simulink model "main_vehicle_model"  (R2023b)
settings: Solver=FixedStepAuto  StartTime=0.0  StopTime=999  RelTol=1e-3  EnableMultiTasking=on
libraries: mbedblockslib x22, mcbcontrolslib x3, slpidlib x1, raspberrypiIMUsensorslib x1, simulink x1
settings Model: SimulationMode=external  ExtModeTrigDuration=10  Creator=Aidan  LastModifiedBy=Aidan
settings SolverCC: AutoInsertRateTranBlk=on
settings OptimizationCC: EnhancedBackFolding=on  PassReuseOutputArgsAs=Individual arguments  ZeroExternalMemoryAtStartup=off  ZeroInternalMemoryAtStartup=off  MaxStackSize=64  OptimizeBlockOrder=speed  DifferentSizesBufferReuse=on  OptimizationCustomize=off  EfficientTunableParamExpr=on
settings DebuggingCC: ParameterTunabilityLossMsg=error
settings HardwareCC: ProdBitPerPointer=32  ProdBitPerSizeT=32  ProdBitPerPtrDiffT=32  ProdLargestAtomicInteger=Long  ProdLargestAtomicFloat=Double  ProdWordSize=32  ProdLongLongMode=on  ProdHWDeviceType=ARM Compatible->ARM Cortex
settings SFSimCC: MATLABDynamicMemAlloc=off
settings RTWCC: Description=Embedded Coder  SystemTargetFile=ert.tlc  HardwareBoard=STM32 Nucleo F746ZG  TemplateMakefile=ert_default_tmf  Toolchain=GNU Tools for ARM Embedded Processors
settings CodeAppCC: ForceParamTrailComments=on  IgnoreCustomStorageClasses=off  OperatorAnnotations=on  SimulinkDataObjDesc=on  SFDataObjDesc=on  InsertBlockDesc=on
settings ERTTargetCC: SupportContinuousTime=on  ExtMode=on  ExtModeTransport=3  ExtModeStaticAlloc=on  ExtModeStaticAllocSize=2000  ExtModeMexFile=ext_xcp  ExtModeMexArgs=1 10 115200  ExtModeIntrfLevel=Level2 - Open

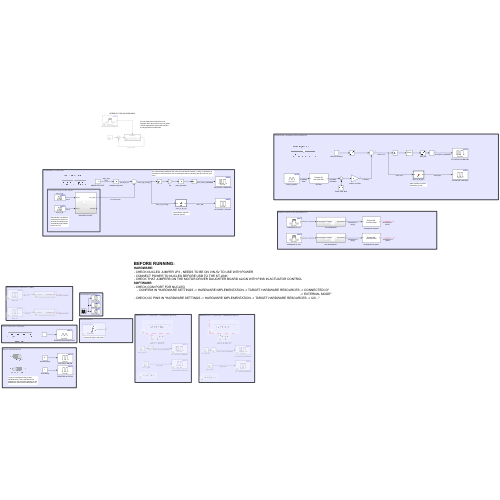
[thumbnail: Simulink's stored preview of the top-level diagram]
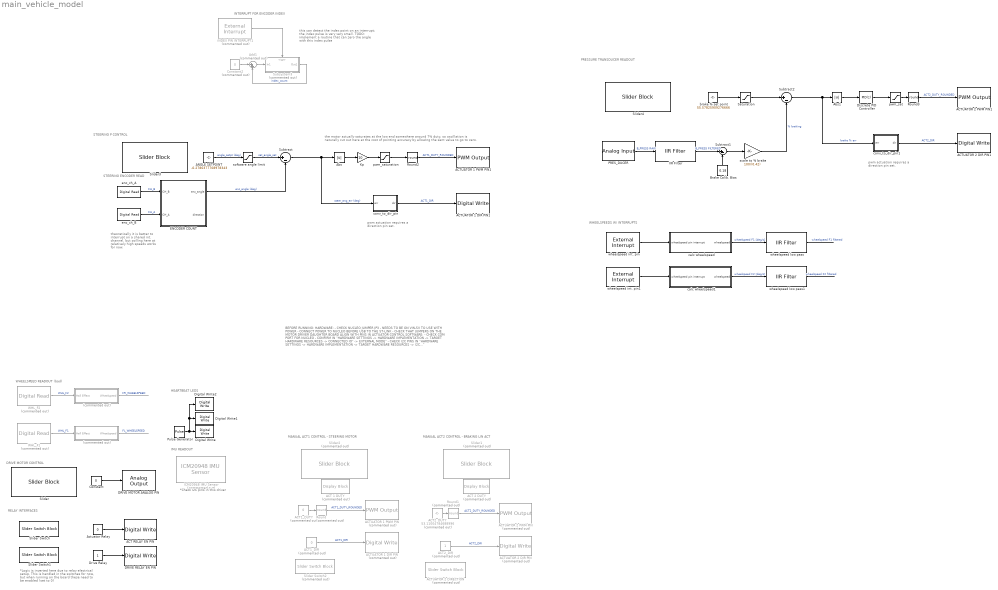
== system main_vehicle_model ==
  note: WHEELSPEEDS W/ INTERRUPTS
  note: this can detect the index point on an interrupt; the index pulse is very very small.
      | TODO: implement a routine that can zero the angle with this index pulse
  note: the motor actually saturates at the low end somewhere around 7% duty, so oscillation is naturally cut out here at the cost of pointing accuracy by allowing the sent value to go to zero.
  note: STEERING P CONTROL
  note: STEERING ENCODER READ
  note: pwm actuation requires a direction pin set.
  note: theoretically it is better to interrupt on a shared int. channel, but polling here at relatively high speeds works for now.
  note: *Check I2C pins in this driver
  note: *Logic is inverted here due to relay electrical setup. This is handled in the switches for now, but when running on the board these need to be enabled (set to 0)
  note: MANUAL ACT2 CONTROL - BRAKING LIN ACT
  note: MANUAL ACT1 CONTROL - STEERING MOTOR
  note: BEFORE RUNNING:
      | HARDWARE:
      | - CHECK NUCLEO JUMPER JP3 - NEEDS TO BE ON VIN-5V TO USE WITH POWER
      | - CONNECT POWER TO NUCLEO BEFORE USB TO THE ST-LINK
      | - CHECK THAT JUMPERS ON THE MOTOR DRIVER DAUGHTER BOARD ALIGN WITH PINS IN ACTUATOR CONTROL
      | SOFTWARE:
      | - CHECK COM PORT FOR NUCLEO
      | - CONFIRM IN "HARDWARE SETTINGS -> HARDWARE IMPLEMENTATION -> TARGET HARDWARE RESOURCES -> CONNECTED IO"
      | -> EXTERNAL MODE"
      | - CHECK I2C PINS IN "HARDWARE SETTINGS -> HARDWARE IMPLEMENTATION -> TARGET HARDWARE RESOURCES -> I2C..."
  note: DRIVE MOTOR CONTROL
  note: RELAY INTERFACES
  note: HEARTBEAT LEDS
  note: PRESSURE TRANSDUCER READOUT
  note: WHEELSPEED READOUT (bad)
  note: IMU READOUT
  note: INTERRUPT FOR ENCODER INDEX
  note: pwm actuation requires a direction pin set.
  " " : Subsystem  Commented=on
  "  " : Subsystem  Commented=on
  ACT 1 DUTY : DisplayBlock  Commented=on  LabelPosition=Hide  Transparency=1
  ACT 2 DUTY : DisplayBlock  Commented=on  LabelPosition=Hide  Transparency=1
  ACT RELAY EN PIN : mbedblockslib/Digital Write  Pin=A1  Direction=output
      settings: LibrarySourceBlock=stmnucleorootlib/Common/Digital Write
  ACT1_DIR : Constant  Commented=on  Value=0
  ACT1_DUTY : Constant  Commented=on  Value=0
  ACT2_DIR : Constant  Commented=on
  ACT2_DUTY : Constant  Commented=on  Value=53.11004784688996
  ACTUATOR 1 DIR PIN : mbedblockslib/Digital Write  Commented=on  Pin=D2  Direction=output
      settings: LibrarySourceBlock=stmnucleorootlib/Common/Digital Write
  ACTUATOR 1 DIR PIN1 : mbedblockslib/Digital Write  Pin=D2  Direction=output
      settings: LibrarySourceBlock=stmnucleorootlib/Common/Digital Write
  ACTUATOR 1 PWM PIN : mbedblockslib/PWM Output  Commented=on  Pin=D3  EnableInputFrequency=off  InitialFrequency=20000  InitialDutyCycle=50  NotificationType=None
      settings: LibrarySourceBlock=stmnucleorootlib/Common/PWM Output
  ACTUATOR 1 PWM PIN1 : mbedblockslib/PWM Output  Pin=D3  EnableInputFrequency=off  InitialFrequency=20000  InitialDutyCycle=0  NotificationType=None
      settings: LibrarySourceBlock=stmnucleorootlib/Common/PWM Output
  ACTUATOR 2 DIR PIN : mbedblockslib/Digital Write  Commented=on  Pin=D7  Direction=output
      settings: LibrarySourceBlock=stmnucleorootlib/Common/Digital Write
  ACTUATOR 2 DIR PIN1 : mbedblockslib/Digital Write  Pin=D7  Direction=output
      settings: LibrarySourceBlock=stmnucleorootlib/Common/Digital Write
  ACTUATOR 2 DIRECTION : SliderSwitchBlock  Commented=on
      settings: Values={{'OUT', 'IN'}, [0 1]}
  ACTUATOR 2 PWM PIN : mbedblockslib/PWM Output  Commented=on  Pin=D11  EnableInputFrequency=off  InitialFrequency=20000  InitialDutyCycle=50  NotificationType=None
      settings: LibrarySourceBlock=stmnucleorootlib/Common/PWM Output
  ACTUATOR 2 PWM PIN1 : mbedblockslib/PWM Output  Pin=D11  EnableInputFrequency=off  InitialFrequency=20000  InitialDutyCycle=50  NotificationType=None
      settings: LibrarySourceBlock=stmnucleorootlib/Common/PWM Output
  ANGLE SETPOINT : Constant  Value=-0.2786377708978343
  Abs : Abs  SaturateOnIntegerOverflow=off
  Abs1 : Abs  SaturateOnIntegerOverflow=off
  Actuator Relay : Constant  Value=0  SampleTime=0.01
  Add1 : Sum  Commented=on  Inputs=|++
  Brake Calib. Bias : Constant  Value=0.18
  Constant : Constant  Value=0  SampleTime=0.01
  Constant2 : Constant  Commented=on  Value=0
  DRIVE MOTOR ANALOG PIN : mbedblockslib/Analog Output  Pin=D13
      settings: LibrarySourceBlock=stmnucleorootlib/Common/Analog Output
  DRIVE RELAY EN PIN : mbedblockslib/Digital Write  Pin=A0  Direction=output
      settings: LibrarySourceBlock=stmnucleorootlib/Common/Digital Write
  Digital Write : mbedblockslib/Digital Write  Pin=PB_7  Direction=output
  Digital Write1 : mbedblockslib/Digital Write  Pin=PB_14  Direction=output
  Digital Write2 : mbedblockslib/Digital Write  Pin=PB_0  Direction=output
  Discrete PID Controller : slpidlib/PID Controller  Controller=PID  Form=Parallel  TimeDomain=Discrete-time  UseExternalTs=off  SampleTime=-1  IntegratorMethod=Forward Euler  FilterMethod=Forward Euler  ControllerParametersSource=internal  P=10  I=5  UseKiTs=off  D=0.0  N=100  UseFilter=on  TunerSelectOption=Transfer Function Based (PID Tuner App)  InitialConditionSource=internal  InitialConditionForIntegrator=0  InitialConditionForFilter=0  DifferentiatorICPrevScaledInput=0  ExternalReset=none  TrackingMode=off  Kt=1  LimitOutput=off  SatLimitsSource=internal  UpperSaturationLimit=inf  LowerSaturationLimit=-inf  LinearizeAsGain=off  AntiWindupMode=none  Kb=1  LimitIntegrator=off  UpperIntegratorSaturationLimit=inf  LowerIntegratorSaturationLimit=-inf  POutMin=[]  POutMax=[]  IOutMin=[]  IOutMax=[]  DOutMin=[]  DOutMax=[]  NOutMin=[]  NOutMax=[]  SumOutMin=[]  SumOutMax=[]  SaturationOutMin=[]  SaturationOutMax=[]  PParamMin=[]  PParamMax=[]  IParamMin=[]  IParamMax=[]  DParamMin=[]  DParamMax=[]  NParamMin=[]  NParamMax=[]  KbParamMin=[]  KbParamMax=[]  KtParamMin=[]  KtParamMax=[]  KbOutMin=[]  KbOutMax=[]  KtOutMin=[]  KtOutMax=[]  IntegratorOutMin=[]  IntegratorOutMax=[]  FilterOutMin=[]  FilterOutMax=[]  SumI1OutMin=[]  SumI1OutMax=[]  SumI2OutMin=[]  SumI2OutMax=[]  SumI3OutMin=[]  SumI3OutMax=[]  SumI4OutMin=[]  SumI4OutMax=[]  SumDOutMin=[]  SumDOutMax=[]  DifferentiatorOutMin=[]  DifferentiatorOutMax=[]  FilterDiffOutCoefMin=[]  FilterDiffOutCoefMax=[]  ReciprocalOutMin=[]  ReciprocalOutMax=[]  SumDenOutMin=[]  SumDenOutMax=[]  SumNumOutMin=[]  SumNumOutMax=[]  DivideOutMin=[]  DivideOutMax=[]  UdiffTsProdOutMin=[]  UdiffTsProdOutMax=[]  NTsProdOutMin=[]  NTsProdOutMax=[]  UintegralTsProdOutMin=[]  UintegralTsProdOutMax=[]  UngainTsProdOutMin=[]  UngainTsProdOutMax=[]  ClampingZeroOutDataTypeStr=Inherit: Inherit via back propagation  ClampingZeroOutMin=[]  ClampingZeroOutMax=[]  FilterDenConstantOutDataTypeStr=Inherit: Inherit via back propagation  FilterDenConstantOutMin=[]  FilterDenConstantOutMax=[]  PCopyOutDataTypeStr=Inherit: Inherit via back propagation  PCopyOutMin=[]  PCopyOutMax=[]  NCopyOutDataTypeStr=Inherit: Inherit via back propagation  NCopyOutMin=[]  NCopyOutMax=[]  IntegratorContinuousStateAttributes=''  IntegratorStateMustResolveToSignalObject=off  IntegratorRTWStateStorageClass=Auto  FilterContinuousStateAttributes=''  FilterStateMustResolveToSignalObject=off  FilterRTWStateStorageClass=Auto  ParallelPVariant=InternalParameters  IdealPVariant=Disabled  IVariant=InternalParameters  DVariant=InternalParameters  IntegratorVariant=Discrete  SatVariant=Disabled  AWVariant=Passthrough  PCopyVariant=Disabled  TRVariant=Disabled  FdbkBlocksVariant=Forward  IdealPFdbkVariant=Disabled  SatFdbkVariant=Disabled  DerivativeFilterVariant=ForwardEulerFilter  NVariant=InternalParameters  NCopyVariant=Disabled  FilterICVariant=InternalICsFilter  IntegratorICVariant=InternalICs  ExternalResetVariant=Disabled  TRSumVariant=Passthrough  SumFdbkVariant=Disabled  SumVariant=Sum_PID  TsampFilterVariant=InternalTs  TsampNgainVariant=Passthrough  TsampIntegralVariant=Disabled_SignalSpec  ExternalSaturationOutDataTypeStr=Inherit: Same as second input
      settings: LibrarySourceBlock=hdlsllib/Discrete/Discrete PID Controller
  Drive Relay : Constant
  ENCODER COUNT : Subsystem
  ICM20948 IMU Sensor : raspberrypiIMUsensorslib/ICM20948 IMU Sensor  Commented=on  I2CModule=0  I2CAddress=0x69  BitRate=1000000  EnableDRDY=off  InterruptType=Active high  IsActiveAccel=on  IsActiveGyro=off  IsActiveMag=off  IsActiveTemp=off  IsActiveStatus=off  IsActiveTimeStamp=off  AccelerometerRange=+/-2g  AccelerometerODR=1125  AccelerometerBW=23.9 Hz  GyroscopeRange=+/-250 dps  GyroscopeODR=1125  GyroscopeBW=23.9 Hz  MagnetometerODR=100 Hz  TemperatureBW=34.1 Hz  DataType=double  SampleTime=0.1  QueueSizeFactor=3
  IIR Filter : mcbcontrolslib/IIR Filter  VariantControl=Low Pass Filter  VariantSelect=Low-pass  Filter_constant=0.01  advancedSettings=on  Ts=50e-6  cutOff_freq=32.1525
      settings: LibrarySourceBlock=mcblib/Signal Management/IIR Filter
  Kp : Gain  Gain=10
  PRES_DUCER : mbedblockslib/Analog Input  Pin=D13  ReadResultsOnly=off  ConversionTriggerSource=Software  ExternalTriggerType=uint32( 0 )  OutputDataType=double  EnableConversionCompleteNotify=off  EnableOuputStatus=off  SampleTime=0.001
      settings: LibrarySourceBlock=stmnucleorootlib/Common/Analog Input
  Pulse Generator : DiscretePulseGenerator  PulseType=Time based  Period=.5  PulseWidth=50  SampleTime=0.1
  Round : Rounding  Commented=on  Operator=round
  Round1 : Rounding  Commented=on  Operator=round
  Round2 : Rounding  Operator=round
  Round3 : Rounding  Operator=round
  Saturation : Saturate  UpperLimit=100  LowerLimit=0
  Slider : SliderBlock  LabelPosition=Bottom  ScaleMax=1  TickInterval=.25
  Slider Switch : SliderSwitchBlock  LabelPosition=Bottom
      settings: Values={{'Off', 'On'}, [1 0]}
  Slider Switch1 : SliderSwitchBlock  LabelPosition=Bottom
      settings: Values={{'Off', 'On'}, [1 0]}
  Slider Switch2 : SliderSwitchBlock  Commented=on
      settings: Values={{'Off', 'On'}, [0 1]}
  Slider1 : SliderBlock  Commented=on
  Slider2 : SliderBlock  Commented=on
  Slider3 : SliderBlock  ScaleMin=-30  ScaleMax=30
  Slider4 : SliderBlock
  Subsystem3 : Subsystem  Commented=on
  Subtract : Sum  Inputs=|+-
  Subtract1 : Sum  Inputs=|+-
  Subtract2 : Sum  Inputs=|+-
  WHL_F1 : mbedblockslib/Digital Read  Commented=on  Pin=D0  Direction=input  SampleTime=-1
      settings: LibrarySourceBlock=stmnucleorootlib/Common/Digital Read
  WHL_F2 : mbedblockslib/Digital Read  Commented=on  Pin=D1  Direction=input  SampleTime=-1
      settings: LibrarySourceBlock=stmnucleorootlib/Common/Digital Read
  brake % set point : Constant  Value=55.57825909276666
  calc wheelspeed : Subsystem
  calc wheelspeed1 : Subsystem
  conv_to_dir_pin : MATLAB Function  TreatAsAtomicUnit=on
  conv_to_dir_pin1 : MATLAB Function  TreatAsAtomicUnit=on
  enc_ch_A : mbedblockslib/Digital Read  Pin=A4  Direction=input  SampleTime=0.00001
      settings: LibrarySourceBlock=stmnucleorootlib/Common/Digital Read
  enc_ch_B : mbedblockslib/Digital Read  Pin=A5  Direction=input  SampleTime=0.00001
      settings: LibrarySourceBlock=stmnucleorootlib/Common/Digital Read
  iNDEX PIN INTERRUPT1 : mbedblockslib/External Interrupt  Commented=on  Pin=A3  Mode=Pull-down  EdgeSelection=Rising  VectorFcnCallOutput=off  SimulationInput=off  InitialPinStatus=false  BlockPlatform=nucleo
      settings: LibrarySourceBlock=stmnucleorootlib/Common/External Interrupt
  pwm_sat : Saturate  UpperLimit=100  LowerLimit=0
  pwm_saturation : Saturate  UpperLimit=100  LowerLimit=0
  scale to % brake : Gain  Gain=100/(0.42)
  software angle limit : Saturate  UpperLimit=33  LowerLimit=-33
  wheelspeed int. pin : mbedblockslib/External Interrupt  Pin=D1  Mode=Pull-down  EdgeSelection=Rising  VectorFcnCallOutput=off  SimulationInput=off  InitialPinStatus=false  BlockPlatform=nucleo
      settings: LibrarySourceBlock=stmnucleorootlib/Common/External Interrupt
  wheelspeed int. pin1 : mbedblockslib/External Interrupt  Pin=D0  Mode=Pull-down  EdgeSelection=Rising  VectorFcnCallOutput=off  SimulationInput=off  InitialPinStatus=false  BlockPlatform=nucleo
      settings: LibrarySourceBlock=stmnucleorootlib/Common/External Interrupt
  wheelspeed low pass : mcbcontrolslib/IIR Filter  VariantControl=Low Pass Filter  VariantSelect=Low-pass  Filter_constant=0.1  advancedSettings=on  Ts=50e-3  cutOff_freq=0.35368
      settings: LibrarySourceBlock=mcblib/Signal Management/IIR Filter
  wheelspeed low pass1 : mcbcontrolslib/IIR Filter  VariantControl=Low Pass Filter  VariantSelect=Low-pass  Filter_constant=0.1  advancedSettings=on  Ts=50e-3  cutOff_freq=0.35368
      settings: LibrarySourceBlock=mcblib/Signal Management/IIR Filter
  wires:
  Actuator Relay/1 -> ACT RELAY EN PIN/1
  Drive Relay/1 -> DRIVE RELAY EN PIN/1
  Constant/1 -> DRIVE MOTOR ANALOG PIN/1
  Pulse Generator/1 -> Digital Write2/1, Digital Write1/1, Digital Write/1
  WHL_F1/1 -> "  "/1(Hall Effect)  "WHL_F1"
  ACT1_DIR/1 -> ACTUATOR 1 DIR PIN/1  "ACT1_DIR"
  ACT1_DUTY/1 -> Round/1
  Round/1 -> ACTUATOR 1 PWM PIN/1  "ACT1_DUTY_ROUNDED"
  ACT2_DIR/1 -> ACTUATOR 2 DIR PIN/1  "ACT2_DIR"
  Round1/1 -> ACTUATOR 2 PWM PIN/1  "ACT2_DUTY_ROUNDED"
  ACT2_DUTY/1 -> Round1/1
  WHL_F2/1 -> " "/1(Hall Effect)  "WHL_F2"
  PRES_DUCER/1 -> IIR Filter/1  "B_PRESS RAW"
  enc_ch_A/1 -> ENCODER COUNT/1(CH_B)  "CH_B"
  enc_ch_B/1 -> ENCODER COUNT/2(CH_A)  "CH_A"
  ENCODER COUNT/1(enc_angle) -> Subtract/2  "enc_angle (deg)"
  Kp/1 -> pwm_saturation/1
  conv_to_dir_pin/1(dir) -> ACTUATOR 1 DIR PIN1/1  "ACT1_DIR"
  Round2/1 -> ACTUATOR 1 PWM PIN1/1  "ACT1_DUTY_ROUNDED"
  ANGLE SETPOINT/1 -> software angle limit/1  "angle_setpt (deg)"
  Subtract/1 -> conv_to_dir_pin/1(err), Abs/1  "steer_ang_err (deg)"
  pwm_saturation/1 -> Round2/1
  Abs/1 -> Kp/1
  software angle limit/1 -> Subtract/1  "sat_angle_set"
  " "/1(Wheelspeed) -> ?  "FR_WHEELSPEED"
  "  "/1(Wheelspeed) -> ?  "FL_WHEELSPEED"
  Subsystem3/1(Out1) -> Add1/2  "index_count"
  iNDEX PIN INTERRUPT1/1 -> Subsystem3/Trigger
  Add1/1 -> Subsystem3/1(In1)
  Constant2/1 -> Add1/1
  IIR Filter/1 -> Subtract1/1  "B_PRESS FILTERED"
  Brake Calib. Bias/1 -> Subtract1/2
  Subtract1/1 -> scale to % brake/1
  scale to % brake/1 -> Subtract2/2  "% braking"
  wheelspeed int. pin/1 -> calc wheelspeed/1(wheelspeed pin interrupt)
  calc wheelspeed/1(wheelspeed) -> wheelspeed low pass/1  "wheelspeed F1 [deg/s]"
  wheelspeed int. pin1/1 -> calc wheelspeed1/1(wheelspeed pin interrupt)
  calc wheelspeed1/1(wheelspeed) -> wheelspeed low pass1/1  "wheelspeed F2 [deg/s]"
  wheelspeed low pass/1 -> ?  "wheelspeed F1 filtered"
  wheelspeed low pass1/1 -> ?  "wheelspeed F2 filtered"
  brake % set point/1 -> Saturation/1
  Saturation/1 -> Subtract2/1
  pwm_sat/1 -> Round3/1
  Round3/1 -> ACTUATOR 2 PWM PIN1/1  "ACT2_DUTY_ROUNDED"
  Subtract2/1 -> conv_to_dir_pin1/1(err), Abs1/1  "brake % err"
  conv_to_dir_pin1/1(dir) -> ACTUATOR 2 DIR PIN1/1  "ACT2_DIR"
  Abs1/1 -> Discrete PID Controller/1
  Discrete PID Controller/1 -> pwm_sat/1

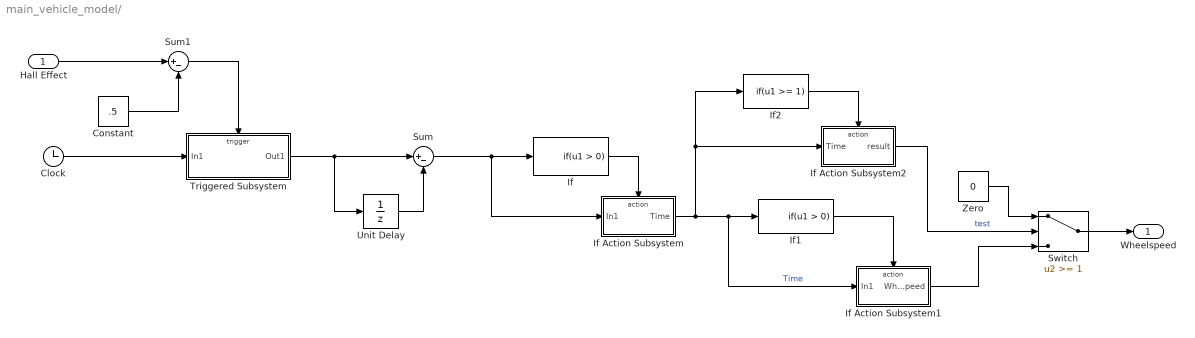
== system main_vehicle_model/  ==
  Hall Effect : Inport
  Clock : Clock
  Constant : Constant  Value=.5
  If : If  ShowElse=off
  If Action Subsystem : Subsystem  TreatAsAtomicUnit=on
  If Action Subsystem1 : Subsystem  TreatAsAtomicUnit=on
  If Action Subsystem2 : Subsystem  TreatAsAtomicUnit=on
  If1 : If  ShowElse=off
  If2 : If  IfExpression=u1 >= 1  ShowElse=off
  Sum : Sum  Inputs=|+-
  Sum1 : Sum  Inputs=|+-
  Switch : Switch  Threshold=1  SaturateOnIntegerOverflow=off  InputSameDT=off
  Triggered Subsystem : Subsystem  TreatAsAtomicUnit=on
  Unit Delay : UnitDelay  SampleTime=-1  HasFrameUpgradeWarning=on
  Zero : Constant  Value=0  OutDataTypeStr=Inherit: Inherit via back propagation
  Wheelspeed : Outport
  wires:
  Sum1/1 -> Triggered Subsystem/Trigger
  If/1 -> If Action Subsystem/Action
  Hall Effect/1 -> Sum1/1
  Clock/1 -> Triggered Subsystem/1(In1)
  Unit Delay/1 -> Sum/2
  Triggered Subsystem/1(Out1) -> Sum/1, Unit Delay/1
  Constant/1 -> Sum1/2
  If Action Subsystem/1(Time) -> If2/1, If Action Subsystem2/1(Time), If Action Subsystem1/1(In1), If1/1  "Time"
  If1/1 -> If Action Subsystem1/Action
  Zero/1 -> Switch/1
  Switch/1 -> Wheelspeed/1
  If Action Subsystem1/1(Wheelspeed) -> Switch/3
  Sum/1 -> If Action Subsystem/1(In1), If/1
  If Action Subsystem2/1(result) -> Switch/2  "test"
  If2/1 -> If Action Subsystem2/Action

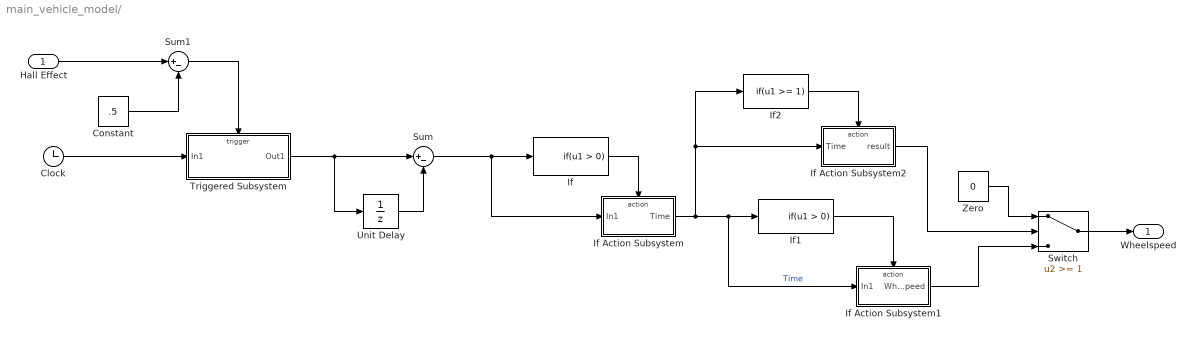
== system main_vehicle_model/   ==
  Hall Effect : Inport
  Clock : Clock
  Constant : Constant  Value=.5
  If : If  ShowElse=off
  If Action Subsystem : Subsystem  TreatAsAtomicUnit=on
  If Action Subsystem1 : Subsystem  TreatAsAtomicUnit=on
  If Action Subsystem2 : Subsystem  TreatAsAtomicUnit=on
  If1 : If  ShowElse=off
  If2 : If  IfExpression=u1 >= 1  ShowElse=off
  Sum : Sum  Inputs=|+-
  Sum1 : Sum  Inputs=|+-
  Switch : Switch  Threshold=1  SaturateOnIntegerOverflow=off  InputSameDT=off
  Triggered Subsystem : Subsystem  TreatAsAtomicUnit=on
  Unit Delay : UnitDelay  SampleTime=-1  HasFrameUpgradeWarning=on
  Zero : Constant  Value=0  OutDataTypeStr=Inherit: Inherit via back propagation
  Wheelspeed : Outport
  wires:
  Sum1/1 -> Triggered Subsystem/Trigger
  If/1 -> If Action Subsystem/Action
  Hall Effect/1 -> Sum1/1
  Clock/1 -> Triggered Subsystem/1(In1)
  Unit Delay/1 -> Sum/2
  Triggered Subsystem/1(Out1) -> Sum/1, Unit Delay/1
  Constant/1 -> Sum1/2
  If Action Subsystem/1(Time) -> If2/1, If Action Subsystem2/1(Time), If Action Subsystem1/1(In1), If1/1  "Time"
  If1/1 -> If Action Subsystem1/Action
  Zero/1 -> Switch/1
  Switch/1 -> Wheelspeed/1
  If Action Subsystem1/1(Wheelspeed) -> Switch/3
  Sum/1 -> If Action Subsystem/1(In1), If/1
  If Action Subsystem2/1(result) -> Switch/2
  If2/1 -> If Action Subsystem2/Action

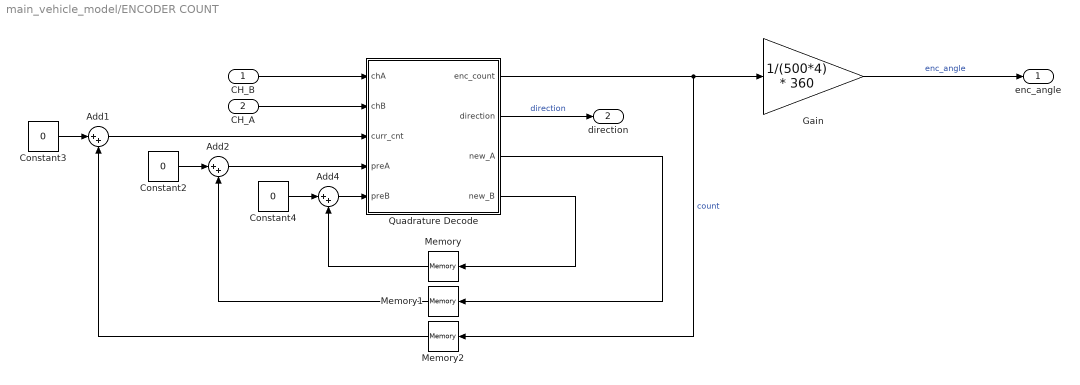
== system main_vehicle_model/ENCODER COUNT ==
  CH_B : Inport
  CH_A : Inport  Port=2
  Add1 : Sum  Inputs=|++
  Add2 : Sum  Inputs=|++
  Add4 : Sum  Inputs=|++
  Constant2 : Constant  Value=0
  Constant3 : Constant  Value=0
  Constant4 : Constant  Value=0
  Gain : Gain  Gain=1/(500*4) * 360
  Memory : Memory
  Memory1 : Memory
  Memory2 : Memory
  Quadrature Decode : MATLAB Function  TreatAsAtomicUnit=on
  enc_angle : Outport
  direction : Outport  Port=2
  wires:
  Add4/1 -> Quadrature Decode/5(preB)
  Constant4/1 -> Add4/1
  CH_A/1 -> Quadrature Decode/2(chB)
  Quadrature Decode/3(new_A) -> Memory1/1
  Quadrature Decode/2(direction) -> direction/1  "direction"
  Memory1/1 -> Add2/2
  Memory/1 -> Add4/2
  Quadrature Decode/1(enc_count) -> Memory2/1, Gain/1  "count"
  Memory2/1 -> Add1/2
  Quadrature Decode/4(new_B) -> Memory/1
  Add1/1 -> Quadrature Decode/3(curr_cnt)
  Constant3/1 -> Add1/1
  Constant2/1 -> Add2/1
  Add2/1 -> Quadrature Decode/4(preA)
  CH_B/1 -> Quadrature Decode/1(chA)
  Gain/1 -> enc_angle/1  "enc_angle"

== system main_vehicle_model/Subsystem3 ==
  In1 : Inport
  function : TriggerPort  TriggerType=function-call  VariantControl=(inherit)
  Increment Stored Integer : simulink/Additional Math & Discrete/Additional Math: Increment - Decrement/Increment Stored Integer
  Out1 : Outport
  wires:
  Increment Stored Integer/1 -> Out1/1
  In1/1 -> Increment Stored Integer/1

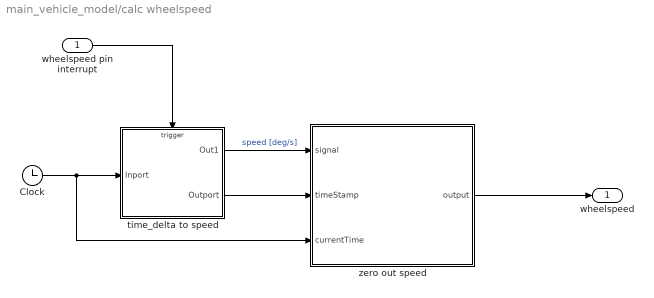
== system main_vehicle_model/calc wheelspeed ==
  wheelspeed pin interrupt : Inport
  Clock : Clock
  time_delta to speed : Subsystem
  zero out speed : MATLAB Function  TreatAsAtomicUnit=on
  wheelspeed : Outport
  wires:
  time_delta to speed/1(Out1) -> zero out speed/1(signal)  "speed [deg/s]"
  Clock/1 -> zero out speed/3(currentTime), time_delta to speed/1(Inport)
  wheelspeed pin interrupt/1 -> time_delta to speed/Trigger
  zero out speed/1(output) -> wheelspeed/1
  time_delta to speed/2(Outport) -> zero out speed/2(timeStamp)

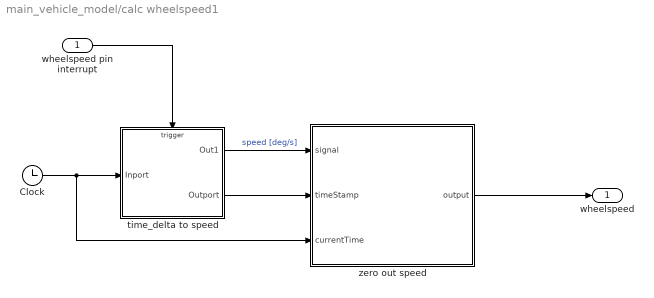
== system main_vehicle_model/calc wheelspeed1 ==
  wheelspeed pin interrupt : Inport
  Clock : Clock
  time_delta to speed : Subsystem
  zero out speed : MATLAB Function  TreatAsAtomicUnit=on
  wheelspeed : Outport
  wires:
  time_delta to speed/1(Out1) -> zero out speed/1(signal)  "speed [deg/s]"
  Clock/1 -> zero out speed/3(currentTime), time_delta to speed/1(Inport)
  wheelspeed pin interrupt/1 -> time_delta to speed/Trigger
  zero out speed/1(output) -> wheelspeed/1
  time_delta to speed/2(Outport) -> zero out speed/2(timeStamp)

== system main_vehicle_model/ /If Action Subsystem ==
  In1 : Inport
  Action Port : ActionPort  ActionPortLabel=if(u1 > 0)
  Time : Outport
  wires:
  In1/1 -> Time/1

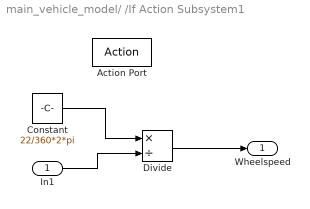
== system main_vehicle_model/ /If Action Subsystem1 ==
  In1 : Inport
  Action Port : ActionPort  ActionPortLabel=if(u1 > 0)
  Constant : Constant  Value=22/360*2*pi
  Divide : Product  Inputs=*/
  Wheelspeed : Outport
  wires:
  In1/1 -> Divide/2
  Divide/1 -> Wheelspeed/1
  Constant/1 -> Divide/1

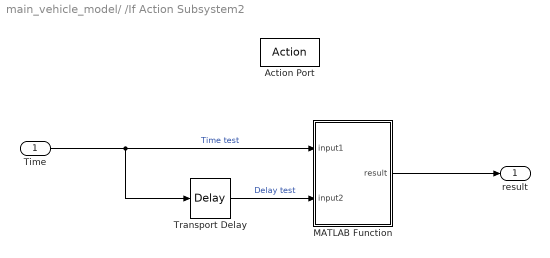
== system main_vehicle_model/ /If Action Subsystem2 ==
  Time : Inport
  Action Port : ActionPort  ActionPortLabel=if(u1 >= 1)
  MATLAB Function : MATLAB Function  TreatAsAtomicUnit=on
  Transport Delay : TransportDelay
  result : Outport
  wires:
  Time/1 -> Transport Delay/1, MATLAB Function/1(input1)  "Time test"
  MATLAB Function/1(result) -> result/1
  Transport Delay/1 -> MATLAB Function/2(input2)  "Delay test"

== system main_vehicle_model/ /Triggered Subsystem ==
  In1 : Inport
  Trigger : TriggerPort  VariantControl=(inherit)
  Out1 : Outport
  wires:
  In1/1 -> Out1/1

== system main_vehicle_model/  /If Action Subsystem ==
  In1 : Inport
  Action Port : ActionPort  ActionPortLabel=if(u1 > 0)
  Time : Outport
  wires:
  In1/1 -> Time/1

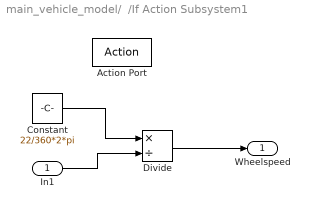
== system main_vehicle_model/  /If Action Subsystem1 ==
  In1 : Inport
  Action Port : ActionPort  ActionPortLabel=if(u1 > 0)
  Constant : Constant  Value=22/360*2*pi
  Divide : Product  Inputs=*/
  Wheelspeed : Outport
  wires:
  In1/1 -> Divide/2
  Divide/1 -> Wheelspeed/1
  Constant/1 -> Divide/1

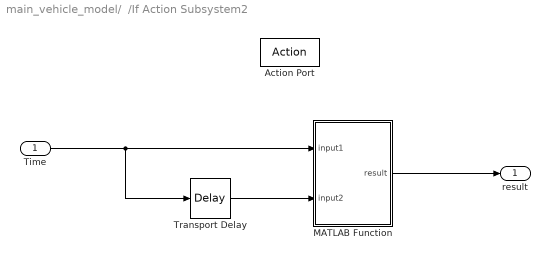
== system main_vehicle_model/  /If Action Subsystem2 ==
  Time : Inport
  Action Port : ActionPort  ActionPortLabel=if(u1 >= 1)
  MATLAB Function : MATLAB Function  TreatAsAtomicUnit=on
  Transport Delay : TransportDelay
  result : Outport
  wires:
  Time/1 -> Transport Delay/1, MATLAB Function/1(input1)
  MATLAB Function/1(result) -> result/1
  Transport Delay/1 -> MATLAB Function/2(input2)

== system main_vehicle_model/  /Triggered Subsystem ==
  In1 : Inport
  Trigger : TriggerPort  VariantControl=(inherit)
  Out1 : Outport
  wires:
  In1/1 -> Out1/1

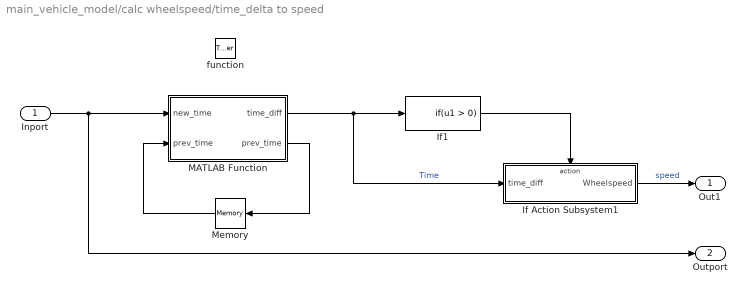
== system main_vehicle_model/calc wheelspeed/time_delta to speed ==
  Inport : Inport
  function : TriggerPort  TriggerType=function-call  VariantControl=(inherit)
  If Action Subsystem1 : Subsystem  TreatAsAtomicUnit=on
  If1 : If  ShowElse=off
  MATLAB Function : MATLAB Function  TreatAsAtomicUnit=on
  Memory : Memory  InheritSampleTime=on
  Out1 : Outport
  Outport : Outport  Port=2
  wires:
  MATLAB Function/2(prev_time) -> Memory/1
  Memory/1 -> MATLAB Function/2("prev_time ")
  If Action Subsystem1/1(Wheelspeed) -> Out1/1  "speed"
  MATLAB Function/1(time_diff) -> If Action Subsystem1/1(time_diff), If1/1  "Time"
  If1/1 -> If Action Subsystem1/Action
  Inport/1 -> Outport/1, MATLAB Function/1(new_time)

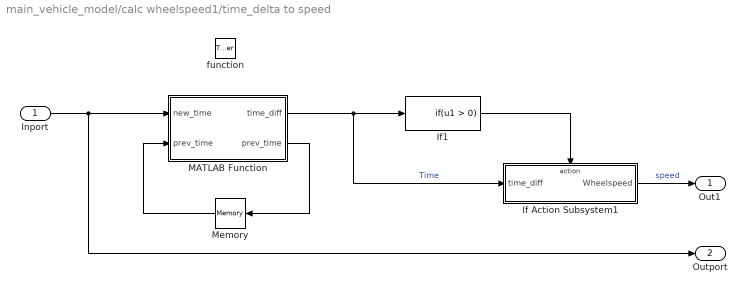
== system main_vehicle_model/calc wheelspeed1/time_delta to speed ==
  Inport : Inport
  function : TriggerPort  TriggerType=function-call  VariantControl=(inherit)
  If Action Subsystem1 : Subsystem  TreatAsAtomicUnit=on
  If1 : If  ShowElse=off
  MATLAB Function : MATLAB Function  TreatAsAtomicUnit=on
  Memory : Memory  InheritSampleTime=on
  Out1 : Outport
  Outport : Outport  Port=2
  wires:
  MATLAB Function/2(prev_time) -> Memory/1
  Memory/1 -> MATLAB Function/2("prev_time ")
  If Action Subsystem1/1(Wheelspeed) -> Out1/1  "speed"
  MATLAB Function/1(time_diff) -> If Action Subsystem1/1(time_diff), If1/1  "Time"
  If1/1 -> If Action Subsystem1/Action
  Inport/1 -> Outport/1, MATLAB Function/1(new_time)

== system main_vehicle_model/calc wheelspeed/time_delta to speed/If Action Subsystem1 ==
  time_diff : Inport
  Action Port : ActionPort  ActionPortLabel=if(u1 > 0)
  Divide : Product  Inputs=*/
  count to radial speed : Constant  Value=22/360*2*pi
  Wheelspeed : Outport
  wires:
  time_diff/1 -> Divide/2
  Divide/1 -> Wheelspeed/1
  count to radial speed/1 -> Divide/1

== system main_vehicle_model/calc wheelspeed1/time_delta to speed/If Action Subsystem1 ==
  time_diff : Inport
  Action Port : ActionPort  ActionPortLabel=if(u1 > 0)
  Divide : Product  Inputs=*/
  count to radial speed : Constant  Value=22/360*2*pi
  Wheelspeed : Outport
  wires:
  time_diff/1 -> Divide/2
  Divide/1 -> Wheelspeed/1
  count to radial speed/1 -> Divide/1

== matlab function main_vehicle_model/conv_to_dir_pin ==
  data: err input; dir output
function dir = fcn(err)

    dir = -1; % invalid state

    if err >=0
        dir = 0;
    elseif err < 0
        dir = 1;
    end
end

== matlab function main_vehicle_model/ENCODER COUNT/Quadrature Decode ==
  data: chA input; enc_count output; direction output; chB input; curr_cnt input; new_A output; new_B output; preA input; preB input
function [enc_count, direction, new_A, new_B] = fcn(chA, chB, curr_cnt, preA, preB)

    New = chA * 2 + chB;
    Old = preA * 2 + preB;

    cmp_arr = [0, -1, 1, 2;
               1, 0, 2, -1;
               -1, 2, 0, 1;
               2, 1, -1, 0];
  
    direction = cmp_arr(Old*4 + New + 1);

    enc_count = curr_cnt + direction;
    new_A = chA;
    new_B = chB;
end

== matlab function main_vehicle_model/ /If Action Subsystem2/MATLAB Function ==
  data: input1 input; result output; input2 input
function result = checkInputs(input1, input2)
% checkInputs - Checks if two inputs are non-zero and equal to each other
%
% Syntax: result = checkInputs(input1, input2)
%
% Inputs:
%    input1 - First input value
%    input2 - Second input value
%
% Outputs:
%    result - Returns 1 if both inputs are non-zero and equal, otherwise returns 0

    if (input1 ~= 0) && (input2 ~= 0) && (input1 == input2)
        result = 1;
    else
        result = 0;
    end
end

== matlab function main_vehicle_model/  /If Action Subsystem2/MATLAB Function ==
  data: input1 input; result output; input2 input
function result = checkInputs(input1, input2)
% checkInputs - Checks if two inputs are non-zero and equal to each other
%
% Syntax: result = checkInputs(input1, input2)
%
% Inputs:
%    input1 - First input value
%    input2 - Second input value
%
% Outputs:
%    result - Returns 1 if both inputs are non-zero and equal, otherwise returns 0

    if (input1 ~= 0) && (input2 ~= 0) && (input1 == input2)
        result = 1;
    else
        result = 0;
    end
end

== matlab function main_vehicle_model/calc wheelspeed/time_delta to speed/MATLAB Function ==
  data: new_time input; prev_time input; time_diff output; prev_time output
function [time_diff, prev_time] = fcn(new_time,prev_time)

if isempty(prev_time)  % Check if prev_time is empty (first execution)
    time_diff = 0;     % Set the time difference to 0 for the first execution
else
    time_diff = new_time - prev_time; % Calculate the time difference
    prev_time = new_time;
end

end

== matlab function main_vehicle_model/calc wheelspeed/zero out speed ==
  data: signal input; output output; timeStamp input; currentTime input
function output = myFunction(signal, timeStamp, currentTime)

if isempty(timeStamp)
    timeStamp = 0;
end

timeDiff = currentTime - timeStamp;

if timeDiff > (1/6)
    output = 0;
else
    output = signal;
end

== matlab function main_vehicle_model/calc wheelspeed1/time_delta to speed/MATLAB Function ==
  data: new_time input; prev_time input; time_diff output; prev_time output
function [time_diff, prev_time] = fcn(new_time,prev_time)

if isempty(prev_time)  % Check if prev_time is empty (first execution)
    time_diff = 0;     % Set the time difference to 0 for the first execution
else
    time_diff = new_time - prev_time; % Calculate the time difference
    prev_time = new_time;
end

end

== matlab function main_vehicle_model/calc wheelspeed1/zero out speed ==
  data: signal input; output output; timeStamp input; currentTime input
function output = myFunction(signal, timeStamp, currentTime)

if isempty(timeStamp)
    timeStamp = 0;
end

timeDiff = currentTime - timeStamp;

if timeDiff > (1/6)
    output = 0;
else
    output = signal;
end

== matlab function main_vehicle_model/conv_to_dir_pin1 ==
  data: err input; dir output
function dir = fcn(err)

    dir = -1; % invalid state

    if err >=0
        dir = 0;
    elseif err < 0
        dir = 1;
    end
end
